simulink model "KITTDynamics"  (R2016b)
settings: Solver=VariableStepAuto  StartTime=0.0  StopTime=8  MaxStep=0.01  RelTol=1e-3
values from neighbouring files (symbols this model uses):
  b = 0.0015    [KITTParameters.m]
  c = 0.02    [KITTParameters.m]
  F_a_max = 80    [KITTParameters.m]
  F_b_max = 000    (= 0)    [KITTParameters.m]
  m = 13    [KITTParameters.m]
settings Model: Creator=sumeetsharma  LastModifiedBy=Sieger

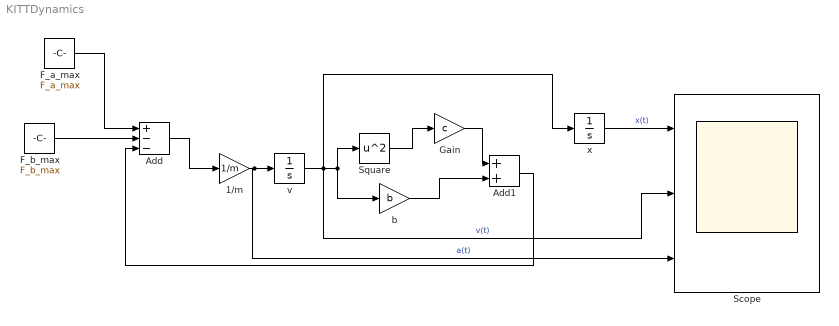
== system KITTDynamics ==
  1/m : Gain  Gain=1/m
  Add : Sum  Inputs=+--
  Add1 : Sum
  F_a_max : Constant  Value=F_a_max
  "F_b_max " : Constant  Value=F_b_max
  Gain : Gain  InitFcn=run KITTParameters.m  Gain=c
  Scope : Scope  NumInputPorts=3
  Square : Math  Operator=square  SaturateOnIntegerOverflow=on
  b : Gain  Gain=b
  v : Integrator  InitialCondition=1
  "x " : Integrator
  wires:
  F_a_max/1 -> Add/1
  "F_b_max "/1 -> Add/2
  Add/1 -> 1/m/1
  1/m/1 -> Scope/3, v/1  "a(t)"
  v/1 -> Scope/2, "x "/1, b/1, Square/1  "v(t)"
  Square/1 -> Gain/1
  Gain/1 -> Add1/1
  b/1 -> Add1/2
  Add1/1 -> Add/3
  "x "/1 -> Scope/1  "x(t)"
